simulink model "TrafficLightSystem_PhyArch_Software"  (R2025b)
settings: Solver=VariableStepAuto  StartTime=0.0  StopTime=10.0  RelTol=1e-3
settings Model: Creator=maric  LastModifiedBy=maric

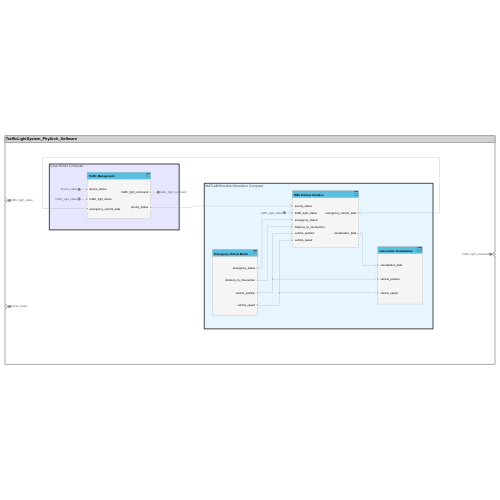
[thumbnail: Simulink's stored preview of the top-level diagram]
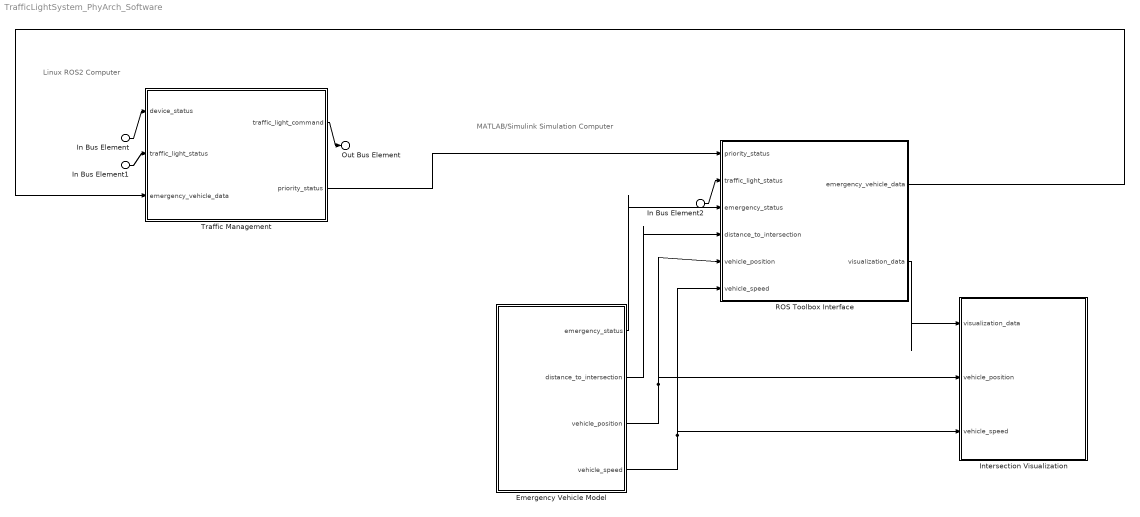
== system TrafficLightSystem_PhyArch_Software ==
  note: MATLAB/Simulink Simulation Computer
  note: Linux ROS2 Computer
  In Bus Element1 : Inport  PortName=traffic_light_status
  In Bus Element2 : Inport  PortName=traffic_light_status
  In Bus Element : Inport  Port=2  PortName=device_status
  Emergency Vehicle Model : Subsystem
      settings: PortSchema="{\"entries\":[{\"content\":{\"headerSize\":26,\"margin\":15,\"minimumSpacing\":25,\"sides\":[{\"content\":{},\"type\":\"ConnectorPlacement.EquallySpacedRectSide\",\"uuid\":\"fc98b1dc-f1c8-4555-a7aa-182a1386029c\"},{\"content\":{\"connectorIds\":[\"Out1\",\"Out4\",\"Out3\",\"Out2\"],\"side\":\"RIGHT\"},\"type\":\"ConnectorPlacement.EquallySpacedRectSide\",\"uuid\":\"c81f0809-b088-4f89-b8c6-4cc559ac91af\"},{\"content\":{\"side\":\"TOP\"},\"type\":\"ConnectorPlacement.EquallySpacedRectSide\",\"uuid\":\"870463db-794f-4bc3-b33a-d9bb69248909\"}]},\"type\":\"ConnectorPlacement.EquallySpacedConnector\",\"uuid\":\"c17be9ea-9773-46b6-98e7-924568083fb3\"}],\"packageUris\":[\"http://schema.mathworks.com/mf0/Connector/R2020b\"],\"version\":\"1.0\"}"
  Intersection Visualization : Subsystem
      settings: PortSchema="{\"entries\":[{\"content\":{\"headerSize\":26,\"margin\":15,\"minimumSpacing\":25,\"sides\":[{\"content\":{\"connectorIds\":[\"In2\",\"In1\",\"In3\"]},\"type\":\"ConnectorPlacement.EquallySpacedRectSide\",\"uuid\":\"fc98b1dc-f1c8-4555-a7aa-182a1386029c\"},{\"content\":{\"side\":\"RIGHT\"},\"type\":\"ConnectorPlacement.EquallySpacedRectSide\",\"uuid\":\"c81f0809-b088-4f89-b8c6-4cc559ac91af\"},{\"content\":{\"side\":\"TOP\"},\"type\":\"ConnectorPlacement.EquallySpacedRectSide\",\"uuid\":\"870463db-794f-4bc3-b33a-d9bb69248909\"}]},\"type\":\"ConnectorPlacement.EquallySpacedConnector\",\"uuid\":\"c17be9ea-9773-46b6-98e7-924568083fb3\"}],\"packageUris\":[\"http://schema.mathworks.com/mf0/Connector/R2020b\"],\"version\":\"1.0\"}"
  ROS Toolbox Interface : Subsystem
      settings: PortSchema="{\"entries\":[{\"content\":{\"headerSize\":26,\"margin\":15,\"minimumSpacing\":25,\"sides\":[{\"content\":{\"connectorIds\":[\"In1\",\"In6\",\"In5\",\"In2\",\"In3\",\"In4\"]},\"type\":\"ConnectorPlacement.EquallySpacedRectSide\",\"uuid\":\"fc98b1dc-f1c8-4555-a7aa-182a1386029c\"},{\"content\":{\"connectorIds\":[\"Out1\",\"Out2\"],\"side\":\"RIGHT\"},\"type\":\"ConnectorPlacement.EquallySpacedRectSide\",\"uuid\":\"c81f0809-b088-4f89-b8c6-4cc559ac91af\"},{\"content\":{\"side\":\"TOP\"},\"type\":\"ConnectorPlacement.EquallySpacedRectSide\",\"uuid\":\"870463db-794f-4bc3-b33a-d9bb69248909\"}]},\"type\":\"ConnectorPlacement.EquallySpacedConnector\",\"uuid\":\"c17be9ea-9773-46b6-98e7-924568083fb3\"}],\"packageUris\":[\"http://schema.mathworks.com/mf0/Connector/R2020b\"],\"version\":\"1.0\"}"
  "Traffic Management " : Subsystem
      settings: PortSchema="{\"entries\":[{\"content\":{\"headerSize\":26,\"margin\":15,\"minimumSpacing\":25,\"sides\":[{\"content\":{\"connectorIds\":[\"In2\",\"In3\",\"In1\"]},\"type\":\"ConnectorPlacement.EquallySpacedRectSide\",\"uuid\":\"fc98b1dc-f1c8-4555-a7aa-182a1386029c\"},{\"content\":{\"connectorIds\":[\"Out2\",\"Out1\"],\"side\":\"RIGHT\"},\"type\":\"ConnectorPlacement.EquallySpacedRectSide\",\"uuid\":\"c81f0809-b088-4f89-b8c6-4cc559ac91af\"},{\"content\":{\"side\":\"TOP\"},\"type\":\"ConnectorPlacement.EquallySpacedRectSide\",\"uuid\":\"870463db-794f-4bc3-b33a-d9bb69248909\"}]},\"type\":\"ConnectorPlacement.EquallySpacedConnector\",\"uuid\":\"c17be9ea-9773-46b6-98e7-924568083fb3\"}],\"packageUris\":[\"http://schema.mathworks.com/mf0/Connector/R2020b\"],\"version\":\"1.0\"}"
  Out Bus Element : Outport  PortName=traffic_light_command
  wires:
  Emergency Vehicle Model/1(emergency_status) -> ROS Toolbox Interface/5(emergency_status)
  ROS Toolbox Interface/2(visualization_data) -> Intersection Visualization/2(visualization_data)
  ROS Toolbox Interface/1(emergency_vehicle_data) -> "Traffic Management "/1(emergency_vehicle_data)
  "Traffic Management "/1(priority_status) -> ROS Toolbox Interface/1(priority_status)
  Emergency Vehicle Model/4(distance_to_intersection) -> ROS Toolbox Interface/2(distance_to_intersection)
  Emergency Vehicle Model/2(vehicle_speed) -> ROS Toolbox Interface/4(vehicle_speed), Intersection Visualization/3(vehicle_speed)
  Emergency Vehicle Model/3(vehicle_position) -> ROS Toolbox Interface/3(vehicle_position), Intersection Visualization/1(vehicle_position)
  In Bus Element/1 -> "Traffic Management "/2(device_status)
  In Bus Element1/1 -> "Traffic Management "/3(traffic_light_status)
  In Bus Element2/1 -> ROS Toolbox Interface/6(traffic_light_status)
  "Traffic Management "/2(traffic_light_command) -> Out Bus Element/1

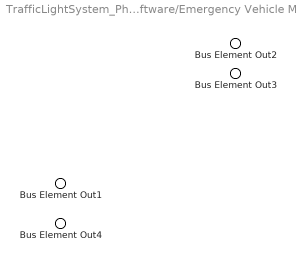
== system TrafficLightSystem_PhyArch_Software/Emergency Vehicle Model ==
  Bus Element Out3 : Outport  PortName=emergency_status
  Bus Element Out2 : Outport  Port=2  PortName=vehicle_speed
  Bus Element Out1 : Outport  Port=3  PortName=vehicle_position
  Bus Element Out4 : Outport  Port=4  PortName=distance_to_intersection

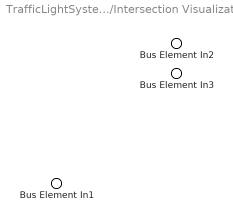
== system TrafficLightSystem_PhyArch_Software/Intersection Visualization ==
  Bus Element In2 : Inport  PortName=vehicle_position
  Bus Element In3 : Inport  Port=2  PortName=visualization_data
  Bus Element In1 : Inport  Port=3  PortName=vehicle_speed

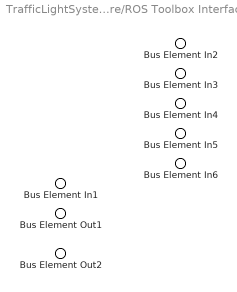
== system TrafficLightSystem_PhyArch_Software/ROS Toolbox Interface ==
  Bus Element In6 : Inport  PortName=priority_status
  Bus Element In5 : Inport  Port=2  PortName=distance_to_intersection
  Bus Element In4 : Inport  Port=3  PortName=vehicle_position
  Bus Element In3 : Inport  Port=4  PortName=vehicle_speed
  Bus Element In2 : Inport  Port=5  PortName=emergency_status
  Bus Element In1 : Inport  Port=6  PortName=traffic_light_status
  Bus Element Out1 : Outport  PortName=emergency_vehicle_data
  Bus Element Out2 : Outport  Port=2  PortName=visualization_data

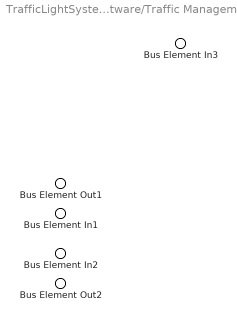
== system TrafficLightSystem_PhyArch_Software/Traffic Management  ==
  Bus Element In1 : Inport  PortName=emergency_vehicle_data
  Bus Element In3 : Inport  Port=2  PortName=device_status
  Bus Element In2 : Inport  Port=3  PortName=traffic_light_status
  Bus Element Out1 : Outport  PortName=priority_status
  Bus Element Out2 : Outport  Port=2  PortName=traffic_light_command
